simulink model "C2_Calculation"  (R2024a)
settings: Solver=VariableStepAuto  StartTime=0.0  StopTime=10.0  RelTol=1e-3
settings Model: Creator=ACER  LastModifiedBy=ACER

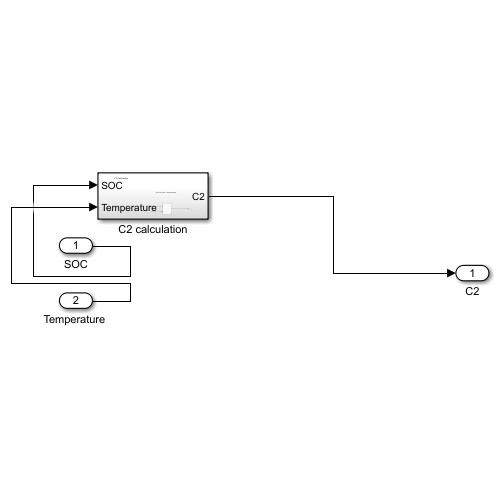
[thumbnail: Simulink's stored preview of the top-level diagram]
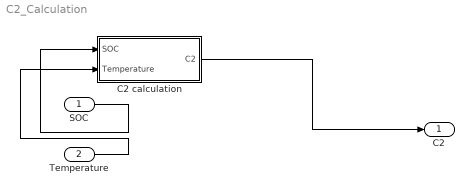
== system C2_Calculation ==
  SOC : Inport
  "Temperature " : Inport  Port=2
  C2 calculation : Subsystem
  C2 : Outport
  wires:
  SOC/1 -> C2 calculation/1(SOC)
  "Temperature "/1 -> C2 calculation/2("Temperature ")
  C2 calculation/1(C2) -> C2/1

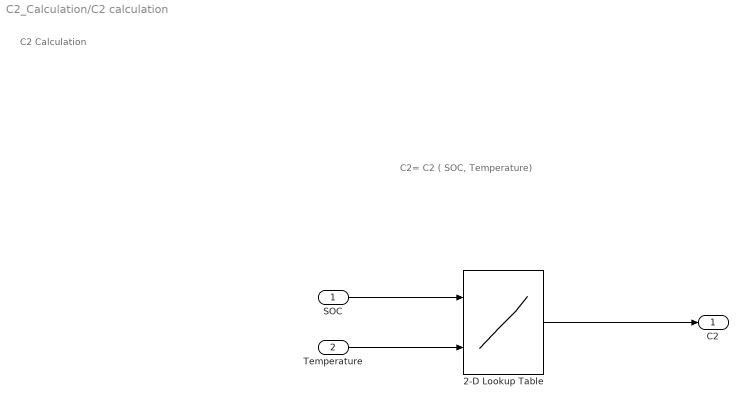
== system C2_Calculation/C2 calculation ==
  note: C2= C2 ( SOC, Temperature)
  note: C2 Calculation
  SOC : Inport
  "Temperature " : Inport  Port=2
  2-D Lookup Table : Lookup_n-D  BreakpointsForDimension1=[1:3]  BreakpointsForDimension2=[1:3]  InternalRulePriority=Speed  RndMeth=Simplest
      settings: InputPortMap=u0,u1
  C2 : Outport
  wires:
  SOC/1 -> 2-D Lookup Table/1
  2-D Lookup Table/1 -> C2/1
  "Temperature "/1 -> 2-D Lookup Table/2
